simulink model "BT1"  (R2019a)
settings: Solver=ode5  StartTime=0.0  StopTime=4  FixedStep=0.001  RelTol=1e-3
libraries: fuzblock x1
settings Model: Creator=ASUS  LastModifiedBy=ASUS

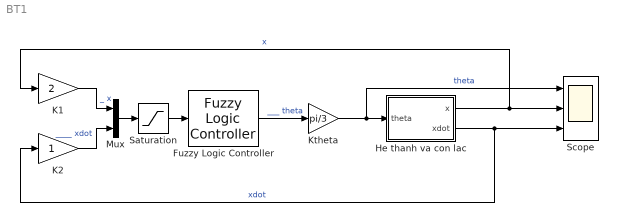
== system BT1 ==
  Fuzzy Logic Controller : fuzblock/Fuzzy Logic  Controller  FIS='bt1.fis'  OutputSampleNumber=101  DataType=double  FuzzifiedInputs=off  RuleFiringStrengths=off  RuleOutputs=off  AggregatedOutputs=off  SimulateUsing=Interpreted execution  OutOfRangeInputValueMessage=warning  NoRuleFiredMessage=warning  EmptyOutputFuzzySetMessage=warning
  He thanh va con lac : Subsystem  mask{m=0.1, R=0.02, g=9.81, J=0.00005, b=0.005, x0=-0.2, xdot0=0.2}
      mask prompts: m "Khoi luong qua bong (kg)"; R "Ban kinh bong"; g "Gia toc trong truong"; J "Momen quan tinh cua qua bong (kgm2)"; b "He so mat sat giua bong va thanh"; x0 "Gia tri dau x0"; xdot0 "Gia tri dau xdot0"
  K1 : Gain  Gain=2
  K2 : Gain
  Ktheta : Gain  Gain=pi/3
  Mux : Mux  Inputs=2
  Saturation : Saturate  UpperLimit=1  LowerLimit=-1
  Scope : Scope  NumInputPorts=3
  wires:
  K1/1 -> Mux/1  "_ x"
  Mux/1 -> Saturation/1
  K2/1 -> Mux/2  "____ xdot"
  Ktheta/1 -> Scope/1, He thanh va con lac/1(theta)  "theta"
  Saturation/1 -> Fuzzy Logic Controller/1
  Fuzzy Logic Controller/1 -> Ktheta/1  "___ theta"
  He thanh va con lac/2(xdot) -> Scope/3, K2/1  "xdot"
  He thanh va con lac/1(x) -> K1/1, Scope/2  "x"

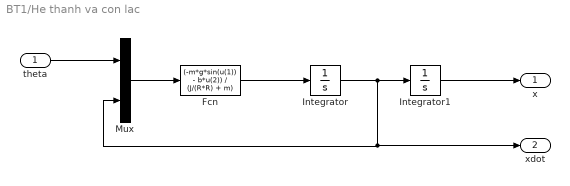
== system BT1/He thanh va con lac ==
  theta : Inport
  Fcn : Fcn  Expr=(-m*g*sin(u(1)) - b*u(2)) / (J/(R*R) + m)
  Integrator : Integrator  InitialCondition=xdot0
  Integrator1 : Integrator  InitialCondition=x0
  Mux : Mux  Inputs=2
  x : Outport
  xdot : Outport  Port=2
  wires:
  theta/1 -> Mux/1
  Fcn/1 -> Integrator/1
  Integrator/1 -> Mux/2, xdot/1, Integrator1/1
  Integrator1/1 -> x/1
  Mux/1 -> Fcn/1
